simulink model "Part1_1"  (R2017a)
settings: Solver=VariableStepAuto  StartTime=0.0  StopTime=10  RelTol=1e-3
libraries: dsparch4 x2, commchan3 x1
settings Model: Creator=mhuynh7  LastModifiedBy=ifaruk

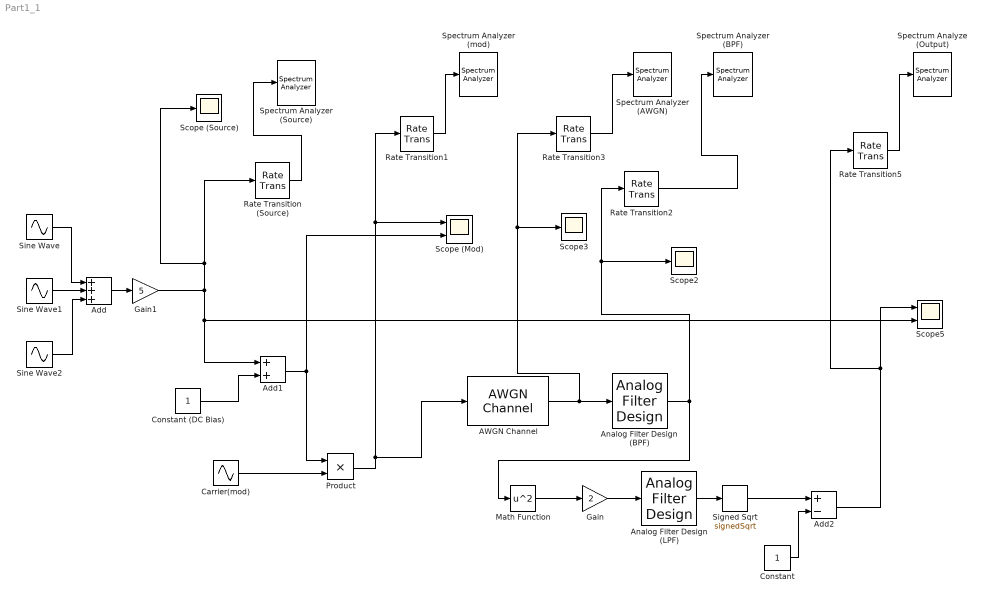
== system Part1_1 ==
  AWGN Channel : commchan3/AWGN Channel  InputProcessing=Columns as channels (frame based)  seed=randseed  noiseMode=Variance from mask  EbNodB=10  EsNodB=10  SNRdB=10  bitsPerSym=1  Ps=1  Tsym=1  variance=0.01
  Add : Sum  Inputs=+++
  Add1 : Sum
  Add2 : Sum  Inputs=+-
  Analog Filter Design (BPF) : dsparch4/Analog Filter Design  method=Butterworth  filttype=Bandpass  N=8  Wlo=20000*pi  Whi=40000*pi  Rp=2  Rs=40
  Analog Filter Design (LPF) : dsparch4/Analog Filter Design  method=Butterworth  filttype=Lowpass  N=8  Wlo=800*2*pi  Whi=80  Rp=2  Rs=40
  Carrier(mod) : Sin  Frequency=30000*pi  Phase=pi/2  SampleTime=0
  Constant : Constant
  Constant (DC Bias) : Constant
  Gain : Gain  Gain=2
  Gain1 : Gain  Gain=5
  Math Function : Math  Operator=square  SaturateOnIntegerOverflow=on
  Product : Product
  Rate Transition (Source) : RateTransition  OutPortSampleTime=1/50000
  Rate Transition{1..3,5} (4 alike) : RateTransition  OutPortSampleTime=1/50000
  Scope (Mod) : Scope  NumInputPorts=2
  Scope (Source) : Scope
  Scope2 : Scope
  Scope3 : Scope
  Scope5 : Scope  NumInputPorts=2
  Signed Sqrt : Sqrt  Operator=signedSqrt  SaturateOnIntegerOverflow=on
  Sine Wave : Sin  Frequency=1000*pi  SampleTime=0
  Sine Wave1 : Sin  Amplitude=3  Frequency=600*pi  SampleTime=0
  Sine Wave2 : Sin  Amplitude=1.5  Frequency=1200*pi  SampleTime=0
  Spectrum Analyze (Output) : SpectrumAnalyzer
  Spectrum Analyzer (AWGN) : SpectrumAnalyzer
  Spectrum Analyzer (BPF) : SpectrumAnalyzer
  Spectrum Analyzer (Source) : SpectrumAnalyzer
  Spectrum Analyzer (mod) : SpectrumAnalyzer
  wires:
  Sine Wave/1 -> Add/1
  Sine Wave1/1 -> Add/2
  Sine Wave2/1 -> Add/3
  Gain1/1 -> Rate Transition (Source)/1, Scope (Source)/1, Add1/1, Scope5/2
  Carrier(mod)/1 -> Product/2
  Rate Transition (Source)/1 -> Spectrum Analyzer (Source)/1
  Product/1 -> AWGN Channel/1, Rate Transition1/1, Scope (Mod)/1
  Rate Transition1/1 -> Spectrum Analyzer (mod)/1
  AWGN Channel/1 -> Scope3/1, Rate Transition3/1, Analog Filter Design (BPF)/1
  Analog Filter Design (BPF)/1 -> Math Function/1, Rate Transition2/1, Scope2/1
  Add2/1 -> Rate Transition5/1, Scope5/1
  Rate Transition5/1 -> Spectrum Analyze (Output)/1
  Rate Transition3/1 -> Spectrum Analyzer (AWGN)/1
  Rate Transition2/1 -> Spectrum Analyzer (BPF)/1
  Constant (DC Bias)/1 -> Add1/2
  Add1/1 -> Scope (Mod)/2, Product/1
  Add/1 -> Gain1/1
  Math Function/1 -> Gain/1
  Gain/1 -> Analog Filter Design (LPF)/1
  Analog Filter Design (LPF)/1 -> Signed Sqrt/1
  Signed Sqrt/1 -> Add2/1
  Constant/1 -> Add2/2
